simulink model "VcScHv"  (R2023b)
settings: Solver=FixedStepDiscrete  StartTime=0.0  StopTime=1  FixedStep=0.01  RelTol=1e-3
model workspace (MAT data in the model file):
  K_VcScHv_BatteryVoltage_Fallback : Simulink.Parameter (value not decoded)
  K_VcScHv_BatteryVoltage_Maximum : Simulink.Parameter (value not decoded)
  K_VcScHv_BatteryVoltage_Minimum : Simulink.Parameter (value not decoded)
  K_VcScHv_BatteryVoltage_Offset : Simulink.Parameter (value not decoded)
  K_VcScHv_BatteryVoltage_Scale : Simulink.Parameter (value not decoded)
  K_VcScHv_BatteryVoltage_Timeout : Simulink.Parameter (value not decoded)
  K_VcScHv_ChargeEnable_Fallback : Simulink.Parameter (value not decoded)
  K_VcScHv_ChargeEnable_Timeout : Simulink.Parameter (value not decoded)
  K_VcScHv_ContactorFeedback_Fallback : Simulink.Parameter (value not decoded)
  K_VcScHv_ContactorFeedback_Timeout : Simulink.Parameter (value not decoded)
  K_VcScHv_CrashSignal_Fallback : Simulink.Parameter (value not decoded)
  K_VcScHv_CrashSignal_Timeout : Simulink.Parameter (value not decoded)
  K_VcScHv_DcLinkVoltage_Fallback : Simulink.Parameter (value not decoded)
  K_VcScHv_DcLinkVoltage_Maximum : Simulink.Parameter (value not decoded)
  K_VcScHv_DcLinkVoltage_Minimum : Simulink.Parameter (value not decoded)
  K_VcScHv_DcLinkVoltage_Offset : Simulink.Parameter (value not decoded)
  K_VcScHv_DcLinkVoltage_Scale : Simulink.Parameter (value not decoded)
  K_VcScHv_DcLinkVoltage_Timeout : Simulink.Parameter (value not decoded)
  K_VcScHv_DriveEnable_Fallback : Simulink.Parameter (value not decoded)
  K_VcScHv_DriveEnable_Timeout : Simulink.Parameter (value not decoded)
  K_VcScHv_IsolationResistance_Fallback : Simulink.Parameter (value not decoded)
  K_VcScHv_IsolationResistance_Maximum : Simulink.Parameter (value not decoded)
  K_VcScHv_IsolationResistance_Minimum : Simulink.Parameter (value not decoded)
  K_VcScHv_IsolationResistance_Offset : Simulink.Parameter (value not decoded)
  K_VcScHv_IsolationResistance_Scale : Simulink.Parameter (value not decoded)
  K_VcScHv_IsolationResistance_Timeout : Simulink.Parameter (value not decoded)
  K_VcScHv_PrechargeFeedback_Fallback : Simulink.Parameter (value not decoded)
  K_VcScHv_PrechargeFeedback_Timeout : Simulink.Parameter (value not decoded)
symbols that are objects in the model workspace (value not decoded): K_VcScHv_BatteryVoltage_Fallback, K_VcScHv_BatteryVoltage_Maximum, K_VcScHv_BatteryVoltage_Minimum, K_VcScHv_BatteryVoltage_Offset, K_VcScHv_BatteryVoltage_Scale, K_VcScHv_BatteryVoltage_Timeout, K_VcScHv_ChargeEnable_Fallback, K_VcScHv_ChargeEnable_Timeout, K_VcScHv_ContactorFeedback_Fallback, K_VcScHv_ContactorFeedback_Timeout, K_VcScHv_CrashSignal_Fallback, K_VcScHv_CrashSignal_Timeout, K_VcScHv_DcLinkVoltage_Fallback, K_VcScHv_DcLinkVoltage_Maximum, K_VcScHv_DcLinkVoltage_Minimum, K_VcScHv_DcLinkVoltage_Offset, K_VcScHv_DcLinkVoltage_Scale, K_VcScHv_DcLinkVoltage_Timeout, K_VcScHv_DriveEnable_Fallback, K_VcScHv_DriveEnable_Timeout, K_VcScHv_IsolationResistance_Fallback, K_VcScHv_IsolationResistance_Maximum, K_VcScHv_IsolationResistance_Minimum, K_VcScHv_IsolationResistance_Offset, K_VcScHv_IsolationResistance_Scale, K_VcScHv_IsolationResistance_Timeout, K_VcScHv_PrechargeFeedback_Fallback, K_VcScHv_PrechargeFeedback_Timeout
libraries: simulink x1
(part 2 of 2)

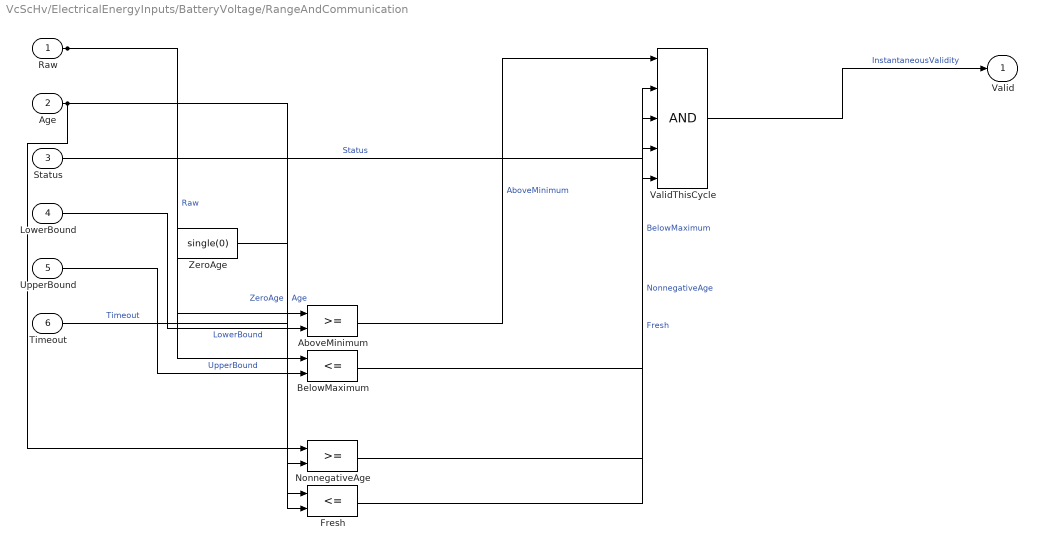
== system VcScHv/ElectricalEnergyInputs/BatteryVoltage/RangeAndCommunication ==
  Raw : Inport
  Age : Inport  Port=2
  Status : Inport  Port=3
  LowerBound : Inport  Port=4
  UpperBound : Inport  Port=5
  Timeout : Inport  Port=6
  AboveMinimum : RelationalOperator  OutDataTypeStr=boolean  RndMeth=Simplest  InputSameDT=off
  BelowMaximum : RelationalOperator  Operator=<=  OutDataTypeStr=boolean  RndMeth=Simplest  InputSameDT=off
  Fresh : RelationalOperator  Operator=<=  OutDataTypeStr=boolean  RndMeth=Simplest  InputSameDT=off
  NonnegativeAge : RelationalOperator  OutDataTypeStr=boolean  RndMeth=Simplest  InputSameDT=off
  ValidThisCycle : Logic  Inputs=5  AllPortsSameDT=off  OutDataTypeStr=boolean
  ZeroAge : Constant  Value=single(0)
  Valid : Outport
  wires:
  Raw/1 -> AboveMinimum/1, BelowMaximum/1  "Raw"
  LowerBound/1 -> AboveMinimum/2  "LowerBound"
  UpperBound/1 -> BelowMaximum/2  "UpperBound"
  Age/1 -> NonnegativeAge/1, Fresh/1  "Age"
  ZeroAge/1 -> NonnegativeAge/2  "ZeroAge"
  Timeout/1 -> Fresh/2  "Timeout"
  AboveMinimum/1 -> ValidThisCycle/1  "AboveMinimum"
  BelowMaximum/1 -> ValidThisCycle/2  "BelowMaximum"
  NonnegativeAge/1 -> ValidThisCycle/3  "NonnegativeAge"
  Fresh/1 -> ValidThisCycle/4  "Fresh"
  Status/1 -> ValidThisCycle/5  "Status"
  ValidThisCycle/1 -> Valid/1  "InstantaneousValidity"

== system VcScHv/ElectricalEnergyInputs/BatteryVoltage/SafeSubstitution ==
  Value : Inport
  Qualified : Inport  Port=2
  Fallback : Inport  Port=3
  SelectSafeValue : Switch  Criteria=u2 ~= 0  SaturateOnIntegerOverflow=off  InputSameDT=off
  SafeValue : Outport
  wires:
  Value/1 -> SelectSafeValue/1  "Value"
  Qualified/1 -> SelectSafeValue/2  "Qualified"
  Fallback/1 -> SelectSafeValue/3  "Fallback"
  SelectSafeValue/1 -> SafeValue/1  "SafeValue"

== system VcScHv/ElectricalEnergyInputs/BatteryVoltage/TemporalQualification ==
  ValidNow : Inport
  Reset : Inport  Port=2
  HistoryInput : Logic  AllPortsSameDT=off  OutDataTypeStr=boolean
  PreviousValid : UnitDelay  InitialCondition=false  SampleTime=-1  HasFrameUpgradeWarning=on
  ResetInactive : Logic  Operator=NOT  AllPortsSameDT=off  OutDataTypeStr=boolean
  TwoConsecutiveValid : Logic  Inputs=3  AllPortsSameDT=off  OutDataTypeStr=boolean
  Qualified : Outport
  wires:
  Reset/1 -> ResetInactive/1  "Reset"
  ValidNow/1 -> HistoryInput/1, TwoConsecutiveValid/1  "TwoConsecutiveValid"
  ResetInactive/1 -> HistoryInput/2, TwoConsecutiveValid/3  "TwoConsecutiveValid"
  HistoryInput/1 -> PreviousValid/1  "ValidityHistory"
  PreviousValid/1 -> TwoConsecutiveValid/2  "TwoConsecutiveValid"
  TwoConsecutiveValid/1 -> Qualified/1  "Qualified"

== system VcScHv/ElectricalEnergyInputs/DcLinkVoltage/EngineeringConversion ==
  Raw : Inport
  Scale : Inport  Port=2
  Offset : Inport  Port=3
  ApplyOffset : Sum
  RawToPhysicalArithmetic : DataTypeConversion  OutDataTypeStr=single  SaturateOnIntegerOverflow=off  RndMeth=Floor
  ScaleRaw : Product
  PhysicalValue : Outport
  wires:
  Raw/1 -> RawToPhysicalArithmetic/1  "TypedRaw"
  RawToPhysicalArithmetic/1 -> ScaleRaw/1  "RawAsSingle"
  Scale/1 -> ScaleRaw/2  "Scale"
  ScaleRaw/1 -> ApplyOffset/1  "Scaled"
  Offset/1 -> ApplyOffset/2  "Offset"
  ApplyOffset/1 -> PhysicalValue/1  "PhysicalValue"

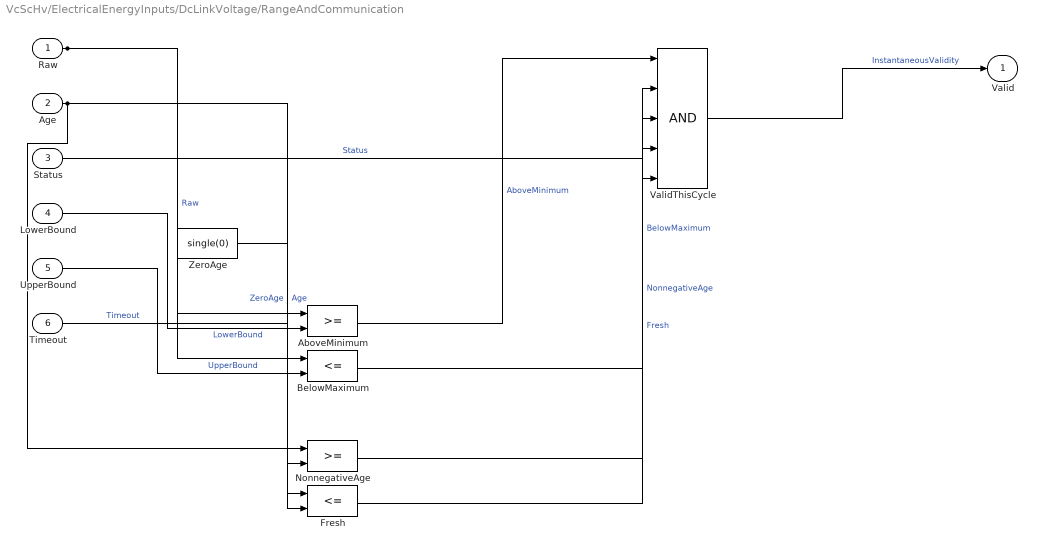
== system VcScHv/ElectricalEnergyInputs/DcLinkVoltage/RangeAndCommunication ==
  Raw : Inport
  Age : Inport  Port=2
  Status : Inport  Port=3
  LowerBound : Inport  Port=4
  UpperBound : Inport  Port=5
  Timeout : Inport  Port=6
  AboveMinimum : RelationalOperator  OutDataTypeStr=boolean  RndMeth=Simplest  InputSameDT=off
  BelowMaximum : RelationalOperator  Operator=<=  OutDataTypeStr=boolean  RndMeth=Simplest  InputSameDT=off
  Fresh : RelationalOperator  Operator=<=  OutDataTypeStr=boolean  RndMeth=Simplest  InputSameDT=off
  NonnegativeAge : RelationalOperator  OutDataTypeStr=boolean  RndMeth=Simplest  InputSameDT=off
  ValidThisCycle : Logic  Inputs=5  AllPortsSameDT=off  OutDataTypeStr=boolean
  ZeroAge : Constant  Value=single(0)
  Valid : Outport
  wires:
  Raw/1 -> AboveMinimum/1, BelowMaximum/1  "Raw"
  LowerBound/1 -> AboveMinimum/2  "LowerBound"
  UpperBound/1 -> BelowMaximum/2  "UpperBound"
  Age/1 -> NonnegativeAge/1, Fresh/1  "Age"
  ZeroAge/1 -> NonnegativeAge/2  "ZeroAge"
  Timeout/1 -> Fresh/2  "Timeout"
  AboveMinimum/1 -> ValidThisCycle/1  "AboveMinimum"
  BelowMaximum/1 -> ValidThisCycle/2  "BelowMaximum"
  NonnegativeAge/1 -> ValidThisCycle/3  "NonnegativeAge"
  Fresh/1 -> ValidThisCycle/4  "Fresh"
  Status/1 -> ValidThisCycle/5  "Status"
  ValidThisCycle/1 -> Valid/1  "InstantaneousValidity"

== system VcScHv/ElectricalEnergyInputs/DcLinkVoltage/SafeSubstitution ==
  Value : Inport
  Qualified : Inport  Port=2
  Fallback : Inport  Port=3
  SelectSafeValue : Switch  Criteria=u2 ~= 0  SaturateOnIntegerOverflow=off  InputSameDT=off
  SafeValue : Outport
  wires:
  Value/1 -> SelectSafeValue/1  "Value"
  Qualified/1 -> SelectSafeValue/2  "Qualified"
  Fallback/1 -> SelectSafeValue/3  "Fallback"
  SelectSafeValue/1 -> SafeValue/1  "SafeValue"

== system VcScHv/ElectricalEnergyInputs/DcLinkVoltage/TemporalQualification ==
  ValidNow : Inport
  Reset : Inport  Port=2
  HistoryInput : Logic  AllPortsSameDT=off  OutDataTypeStr=boolean
  PreviousValid : UnitDelay  InitialCondition=false  SampleTime=-1  HasFrameUpgradeWarning=on
  ResetInactive : Logic  Operator=NOT  AllPortsSameDT=off  OutDataTypeStr=boolean
  TwoConsecutiveValid : Logic  Inputs=3  AllPortsSameDT=off  OutDataTypeStr=boolean
  Qualified : Outport
  wires:
  Reset/1 -> ResetInactive/1  "Reset"
  ValidNow/1 -> HistoryInput/1, TwoConsecutiveValid/1  "TwoConsecutiveValid"
  ResetInactive/1 -> HistoryInput/2, TwoConsecutiveValid/3  "TwoConsecutiveValid"
  HistoryInput/1 -> PreviousValid/1  "ValidityHistory"
  PreviousValid/1 -> TwoConsecutiveValid/2  "TwoConsecutiveValid"
  TwoConsecutiveValid/1 -> Qualified/1  "Qualified"

== system VcScHv/ElectricalEnergyInputs/IsolationResistance/EngineeringConversion ==
  Raw : Inport
  Scale : Inport  Port=2
  Offset : Inport  Port=3
  ApplyOffset : Sum
  RawToPhysicalArithmetic : DataTypeConversion  OutDataTypeStr=single  SaturateOnIntegerOverflow=off  RndMeth=Floor
  ScaleRaw : Product
  PhysicalValue : Outport
  wires:
  Raw/1 -> RawToPhysicalArithmetic/1  "TypedRaw"
  RawToPhysicalArithmetic/1 -> ScaleRaw/1  "RawAsSingle"
  Scale/1 -> ScaleRaw/2  "Scale"
  ScaleRaw/1 -> ApplyOffset/1  "Scaled"
  Offset/1 -> ApplyOffset/2  "Offset"
  ApplyOffset/1 -> PhysicalValue/1  "PhysicalValue"

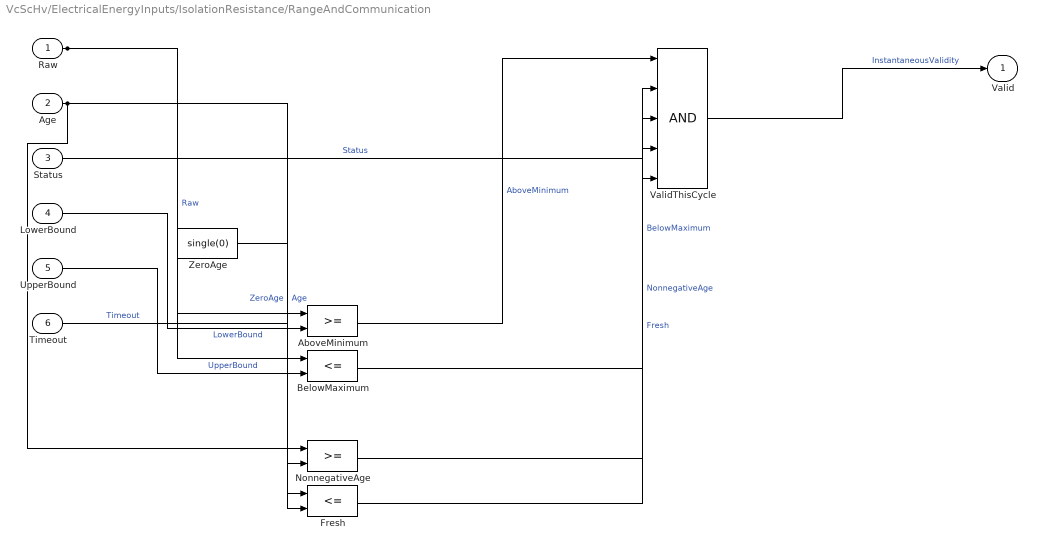
== system VcScHv/ElectricalEnergyInputs/IsolationResistance/RangeAndCommunication ==
  Raw : Inport
  Age : Inport  Port=2
  Status : Inport  Port=3
  LowerBound : Inport  Port=4
  UpperBound : Inport  Port=5
  Timeout : Inport  Port=6
  AboveMinimum : RelationalOperator  OutDataTypeStr=boolean  RndMeth=Simplest  InputSameDT=off
  BelowMaximum : RelationalOperator  Operator=<=  OutDataTypeStr=boolean  RndMeth=Simplest  InputSameDT=off
  Fresh : RelationalOperator  Operator=<=  OutDataTypeStr=boolean  RndMeth=Simplest  InputSameDT=off
  NonnegativeAge : RelationalOperator  OutDataTypeStr=boolean  RndMeth=Simplest  InputSameDT=off
  ValidThisCycle : Logic  Inputs=5  AllPortsSameDT=off  OutDataTypeStr=boolean
  ZeroAge : Constant  Value=single(0)
  Valid : Outport
  wires:
  Raw/1 -> AboveMinimum/1, BelowMaximum/1  "Raw"
  LowerBound/1 -> AboveMinimum/2  "LowerBound"
  UpperBound/1 -> BelowMaximum/2  "UpperBound"
  Age/1 -> NonnegativeAge/1, Fresh/1  "Age"
  ZeroAge/1 -> NonnegativeAge/2  "ZeroAge"
  Timeout/1 -> Fresh/2  "Timeout"
  AboveMinimum/1 -> ValidThisCycle/1  "AboveMinimum"
  BelowMaximum/1 -> ValidThisCycle/2  "BelowMaximum"
  NonnegativeAge/1 -> ValidThisCycle/3  "NonnegativeAge"
  Fresh/1 -> ValidThisCycle/4  "Fresh"
  Status/1 -> ValidThisCycle/5  "Status"
  ValidThisCycle/1 -> Valid/1  "InstantaneousValidity"

== system VcScHv/ElectricalEnergyInputs/IsolationResistance/SafeSubstitution ==
  Value : Inport
  Qualified : Inport  Port=2
  Fallback : Inport  Port=3
  SelectSafeValue : Switch  Criteria=u2 ~= 0  SaturateOnIntegerOverflow=off  InputSameDT=off
  SafeValue : Outport
  wires:
  Value/1 -> SelectSafeValue/1  "Value"
  Qualified/1 -> SelectSafeValue/2  "Qualified"
  Fallback/1 -> SelectSafeValue/3  "Fallback"
  SelectSafeValue/1 -> SafeValue/1  "SafeValue"

== system VcScHv/ElectricalEnergyInputs/IsolationResistance/TemporalQualification ==
  ValidNow : Inport
  Reset : Inport  Port=2
  HistoryInput : Logic  AllPortsSameDT=off  OutDataTypeStr=boolean
  PreviousValid : UnitDelay  InitialCondition=false  SampleTime=-1  HasFrameUpgradeWarning=on
  ResetInactive : Logic  Operator=NOT  AllPortsSameDT=off  OutDataTypeStr=boolean
  TwoConsecutiveValid : Logic  Inputs=3  AllPortsSameDT=off  OutDataTypeStr=boolean
  Qualified : Outport
  wires:
  Reset/1 -> ResetInactive/1  "Reset"
  ValidNow/1 -> HistoryInput/1, TwoConsecutiveValid/1  "TwoConsecutiveValid"
  ResetInactive/1 -> HistoryInput/2, TwoConsecutiveValid/3  "TwoConsecutiveValid"
  HistoryInput/1 -> PreviousValid/1  "ValidityHistory"
  PreviousValid/1 -> TwoConsecutiveValid/2  "TwoConsecutiveValid"
  TwoConsecutiveValid/1 -> Qualified/1  "Qualified"

== matlab function VcScHv/BusinessDecision/HighVoltageSequencer/Implementation ==
  data: in_BatteryVoltage input; out_CommandState output; in_DcLinkVoltage input; in_IsolationResistance input; in_CrashSignal input; in_DriveEnable input; in_ChargeEnable input; in_ContactorFeedback input; in_PrechargeFeedback input; in_valid input; in_reset input; out_ElapsedPrecharge output; out_PrechargeRequest output; out_MainRequest output
function [out_CommandState,out_ElapsedPrecharge,out_PrechargeRequest,out_MainRequest] = component(in_BatteryVoltage,in_DcLinkVoltage,in_IsolationResistance,in_CrashSignal,in_DriveEnable,in_ChargeEnable,in_ContactorFeedback,in_PrechargeFeedback,in_valid,in_reset)
BatteryVoltage=double(in_BatteryVoltage);
DcLinkVoltage=double(in_DcLinkVoltage);
IsolationResistance=double(in_IsolationResistance);
CrashSignal=double(in_CrashSignal);
DriveEnable=double(in_DriveEnable);
ChargeEnable=double(in_ChargeEnable);
ContactorFeedback=double(in_ContactorFeedback);
PrechargeFeedback=double(in_PrechargeFeedback);
valid=double(in_valid);
reset=double(in_reset);
persistent state elapsedTicks
if isempty(state),state=0;elapsedTicks=0;end
requested=DriveEnable~=0 || ChargeEnable~=0;
if reset~=0 || ~requested,state=0;elapsedTicks=0;
elseif valid==0 || IsolationResistance<100000 || CrashSignal~=0,state=3;elapsedTicks=0;
elseif state==0,state=1;elapsedTicks=0;
elseif state==1
 elapsedTicks=elapsedTicks+1;
 if elapsedTicks>50,state=3;
 elseif BatteryVoltage>=100 && DcLinkVoltage>=0.95*BatteryVoltage && PrechargeFeedback~=0,state=2;
 elseif elapsedTicks>=50,state=3;
 end
elseif state==2 && ContactorFeedback==0,state=3;
end
v0=state;v1=elapsedTicks*0.01;v2=double(state==1);v3=double(state==2);
out_CommandState=single(v0);
out_ElapsedPrecharge=single(v1);
out_PrechargeRequest=single(v2);
out_MainRequest=single(v3);
end
